simulink model "Simulink_lab2"  (R2022b)
settings: Solver=VariableStepAuto  StartTime=0.0  StopTime=5  RelTol=1e-3
values from neighbouring files (symbols this model uses):
  A = [0 1 ... (first row only)    [Matlab_.m]    (also in THISISTHEMAINMATLABFIEL.m = A_new)
  B = [0; 239.4]    [Matlab_.m]    (also in THISISTHEMAINMATLABFIEL.m = [B; 0])
  C = [0 1]    [Matlab_.m]    (also in THISISTHEMAINMATLABFIEL.m = [0 0.1 0])
  K1 = K(1)    [Matlab_.m]
  KK = [0 K(2)]    [Matlab_.m]
  L = acker(A',C',observerPoles)    [THISISTHEMAINMATLABFIEL.m]
settings Model: SimulationMode=accelerator  Creator=havso  LastModifiedBy=havso

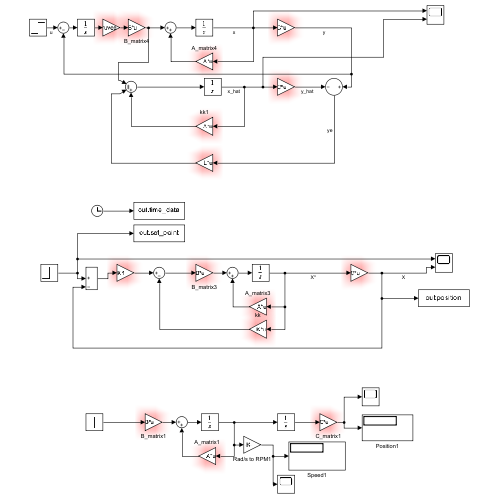
[thumbnail: Simulink's stored preview of the top-level diagram]
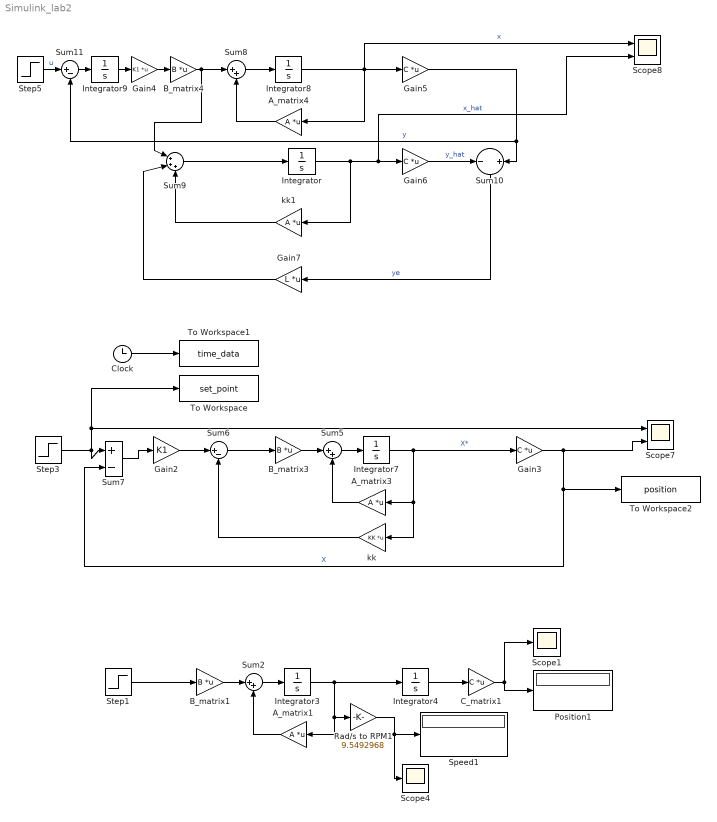
== system Simulink_lab2 ==
  A_matrix1 : Gain  Gain=A  Multiplication=Matrix(K*u)
  A_matrix3 : Gain  Gain=A  Multiplication=Matrix(K*u)
  A_matrix4 : Gain  Gain=A  Multiplication=Matrix(K*u)
  B_matrix1 : Gain  Gain=B  Multiplication=Matrix(K*u)
  B_matrix3 : Gain  Gain=B  Multiplication=Matrix(K*u)
  B_matrix4 : Gain  Gain=B  Multiplication=Matrix(K*u)
  C_matrix1 : Gain  Gain=C  Multiplication=Matrix(K*u)
  Clock : Clock
  Gain2 : Gain  Gain=K1
  Gain3 : Gain  Gain=C  Multiplication=Matrix(K*u)
  Gain4 : Gain  Gain=K1  Multiplication=Matrix(K*u) (u vector)
  Gain5 : Gain  Gain=C  Multiplication=Matrix(K*u)
  Gain6 : Gain  Gain=C  Multiplication=Matrix(K*u)
  Gain7 : Gain  Gain=L  Multiplication=Matrix(K*u)
  Integrator{,3..4,7,9} (5 alike) : Integrator
  Integrator8 : Integrator  InitialCondition=10
  Position1 : Display
  Rad/s to RPM1 : Gain  Gain=9.5492968
  Scope1 : Scope
  Scope4 : Scope
  Scope7 : Scope  NumInputPorts=2
  Scope8 : Scope  NumInputPorts=2
  Speed1 : Display
  Step1 : Step  After=3  SampleTime=0
  Step3 : Step  After=500  SampleTime=0
  Step5 : Step  SampleTime=0
  Sum10 : Sum  Inputs=-||+
  Sum11 : Sum  Inputs=|+-
  Sum2 : Sum  Inputs=|++
  Sum5 : Sum  Inputs=|++
  Sum6 : Sum  Inputs=|+-
  Sum7 : Sum  Inputs=|+-
  Sum8 : Sum  Inputs=|++
  Sum9 : Sum  Inputs=|+++
  To Workspace : ToWorkspace  VariableName=set_point  SampleTime=-1
  To Workspace1 : ToWorkspace  VariableName=time_data  SampleTime=-1
  To Workspace2 : ToWorkspace  VariableName=position  SampleTime=-1
  kk : Gain  Gain=KK  Multiplication=Matrix(K*u)
  kk1 : Gain  Gain=A  Multiplication=Matrix(K*u)
  wires:
  Integrator4/1 -> C_matrix1/1
  C_matrix1/1 -> Scope1/1, Position1/1
  Rad/s to RPM1/1 -> Scope4/1, Speed1/1
  Step1/1 -> B_matrix1/1
  Integrator3/1 -> Rad/s to RPM1/1, A_matrix1/1, Integrator4/1
  B_matrix1/1 -> Sum2/1
  Sum2/1 -> Integrator3/1
  A_matrix1/1 -> Sum2/2
  Sum6/1 -> B_matrix3/1
  Integrator7/1 -> Gain3/1, kk/1, A_matrix3/1  "X*"
  Sum5/1 -> Integrator7/1
  B_matrix3/1 -> Sum5/1
  A_matrix3/1 -> Sum5/2
  kk/1 -> Sum6/2
  Sum7/1 -> Gain2/1
  Step3/1 -> To Workspace/1, Scope7/1, Sum7/1
  Gain2/1 -> Sum6/1
  Clock/1 -> To Workspace1/1
  Gain3/1 -> Scope7/2, To Workspace2/1, Sum7/2  "X"
  Sum8/1 -> Integrator8/1
  A_matrix4/1 -> Sum8/2
  Integrator8/1 -> A_matrix4/1, Scope8/1, Gain5/1  "x"
  B_matrix4/1 -> Sum9/1, Sum8/1
  Gain5/1 -> Sum10/2, Sum11/2  "y"
  Gain6/1 -> Sum10/1  "y_hat"
  kk1/1 -> Sum9/3
  Sum9/1 -> Integrator/1
  Integrator/1 -> Scope8/2, Gain6/1, kk1/1  "x_hat"
  Gain7/1 -> Sum9/2
  Sum10/1 -> Gain7/1  "ye"
  Step5/1 -> Sum11/1  "u"
  Gain4/1 -> B_matrix4/1
  Sum11/1 -> Integrator9/1
  Integrator9/1 -> Gain4/1
